simulink model "Lab7_przygotowanie_2"  (R2022b)
settings: Solver=VariableStepAuto  StartTime=0.0  StopTime=10  RelTol=1e-3
undefined symbols (not defined in the file): Cvp, Cvw, dqg, dTzew, kcp, kcw, kcwp, Kp, L12, M, qg0, t0, Ti, Tp0, Twew0, Tzew0
settings Model: Creator=Dawkin  LastModifiedBy=Dawid
settings DataIOCC: ReturnWorkspaceOutputs=off

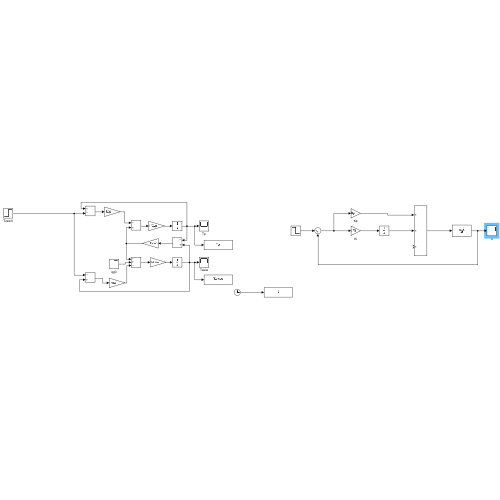
[thumbnail: Simulink's stored preview of the top-level diagram]
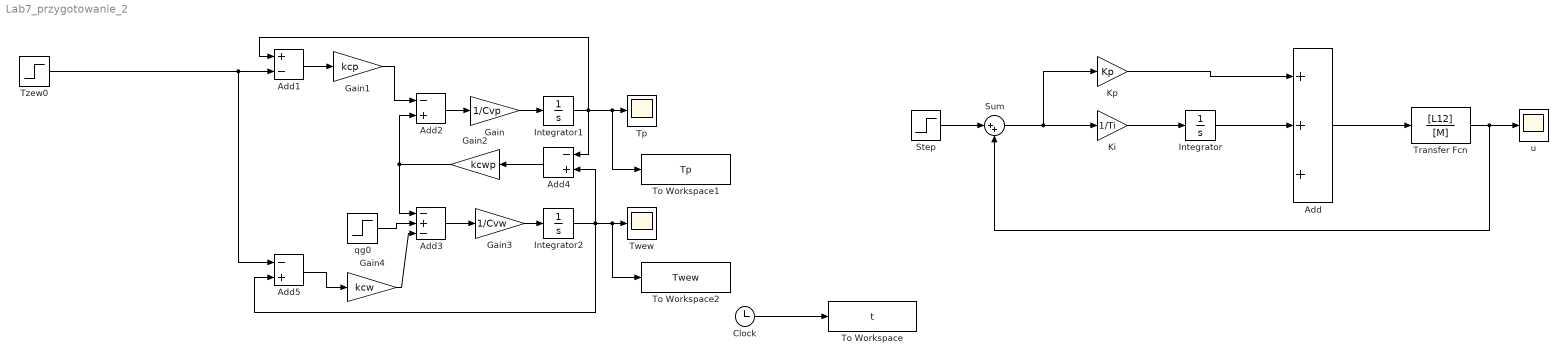
== system Lab7_przygotowanie_2 ==
  Add : Sum  Inputs=+++
  Add1 : Sum  Inputs=+-
  Add2 : Sum  Inputs=-+
  Add3 : Sum  Inputs=-+-
  Add4 : Sum  Inputs=-+
  Add5 : Sum  Inputs=-+
  Clock : Clock
  Gain : Gain  Gain=1/Cvp
  Gain1 : Gain  Gain=kcp
  Gain2 : Gain  Gain=kcwp
  Gain3 : Gain  Gain=1/Cvw
  Gain4 : Gain  Gain=kcw
  Integrator : Integrator
  Integrator1 : Integrator  InitialCondition=Tp0
  Integrator2 : Integrator  InitialCondition=Twew0
  Ki : Gain  Gain=1/Ti
  Kp : Gain  Gain=Kp
  Step : Step  Time=t0  Before=Tp0  SampleTime=0
  Sum : Sum  Inputs=|++
  To Workspace : ToWorkspace  VariableName=t  SaveFormat=Timeseries  SampleTime=-1
  To Workspace1 : ToWorkspace  VariableName=Tp  SampleTime=-1
  To Workspace2 : ToWorkspace  VariableName=Twew  SampleTime=-1
  Tp : Scope
  Transfer Fcn : TransferFcn  Numerator=[L12]  Denominator=[M]
  Twew : Scope
  Tzew0 : Step  Time=t0  Before=Tzew0  After=Tzew0+dTzew  SampleTime=0
  qg0 : Step  Time=t0  Before=qg0  After=qg0+dqg  SampleTime=0
  u : Scope
  wires:
  Step/1 -> Sum/1
  Sum/1 -> Kp/1, Ki/1
  Ki/1 -> Integrator/1
  Kp/1 -> Add/1
  Integrator/1 -> Add/2
  Add/1 -> Transfer Fcn/1
  Transfer Fcn/1 -> Sum/2, u/1
  Gain4/1 -> Add3/3
  Add5/1 -> Gain4/1
  Gain1/1 -> Add2/1
  Add1/1 -> Gain1/1
  Add2/1 -> Gain/1
  Gain/1 -> Integrator1/1
  Add4/1 -> Gain2/1
  Tzew0/1 -> Add1/2, Add5/1
  Integrator2/1 -> Add5/2, Add4/2, To Workspace2/1, Twew/1
  Add3/1 -> Gain3/1
  Integrator1/1 -> To Workspace1/1, Tp/1, Add1/1, Add4/1
  qg0/1 -> Add3/2
  Gain2/1 -> Add2/2, Add3/1
  Gain3/1 -> Integrator2/1
  Clock/1 -> To Workspace/1
